simulink model "IOControls"  (R2019b)
settings: configuration reference "ConfigSet_IOControls_Reference" (kept outside this file)
model workspace (MAT data in the model file):
  SampleTime = 0.05
libraries: IOStateMachinesLib x274, SignalGeneratorsLib x1, simulink x1
(part 9 of 10)

== system IOControls/ForEachVehicle/IOControls/Non-CabControl/PneumaticControls/EPIC ==
  note: States:
      | Isolated
      | Normal
  InputControl : Inport  OutDataTypeStr=Bus: BD_IOControls_In_InputControl
  Initialise : Inport  Port=2
  Bus Selector : BusSelector  OutputSignals=Value,Mode,InitVal,InternalRequest,Inhibit
  EPIC-Toggle : IOStateMachinesLib/Toggle  InitSource=internal  InitState=InitState  OffStateValue=OffStateValue  OnStateValue=OnStateValue
      settings: SourceProductName=IO State Machines
  InputState : Outport  VectorParamsAs1DForOutWhenUnconnected=off
  wires:
  Initialise/1 -> EPIC-Toggle/4
  EPIC-Toggle/1 -> InputState/1
  Bus Selector/5 -> EPIC-Toggle/6  "<Inhibit>"
  Bus Selector/4 -> EPIC-Toggle/5  "<InternalRequest>"
  Bus Selector/3 -> EPIC-Toggle/3  "<InitVal>"
  Bus Selector/2 -> EPIC-Toggle/2  "<Mode>"
  Bus Selector/1 -> EPIC-Toggle/1  "<Value>"
  InputControl/1 -> Bus Selector/1

== system IOControls/ForEachVehicle/IOControls/Non-CabControl/PneumaticControls/Horn1IsolationCock ==
  note: States:
      | Isolated
      | Normal
  InputControl : Inport  OutDataTypeStr=Bus: BD_IOControls_In_InputControl
  Initialise : Inport  Port=2
  Bus Selector : BusSelector  OutputSignals=Value,Mode,InitVal,InternalRequest,Inhibit
  Horn1IsolationCock-Toggle : IOStateMachinesLib/Toggle  InitSource=internal  InitState=InitState  OffStateValue=OffStateValue  OnStateValue=OnStateValue
      settings: SourceProductName=IO State Machines
  InputState : Outport  VectorParamsAs1DForOutWhenUnconnected=off
  wires:
  Initialise/1 -> Horn1IsolationCock-Toggle/4
  Horn1IsolationCock-Toggle/1 -> InputState/1
  Bus Selector/5 -> Horn1IsolationCock-Toggle/6  "<Inhibit>"
  Bus Selector/4 -> Horn1IsolationCock-Toggle/5  "<InternalRequest>"
  Bus Selector/3 -> Horn1IsolationCock-Toggle/3  "<InitVal>"
  Bus Selector/2 -> Horn1IsolationCock-Toggle/2  "<Mode>"
  Bus Selector/1 -> Horn1IsolationCock-Toggle/1  "<Value>"
  InputControl/1 -> Bus Selector/1

== system IOControls/ForEachVehicle/IOControls/Non-CabControl/PneumaticControls/Horn2IsolationCock ==
  note: States:
      | Isolated
      | Normal
  InputControl : Inport  OutDataTypeStr=Bus: BD_IOControls_In_InputControl
  Initialise : Inport  Port=2
  Bus Selector : BusSelector  OutputSignals=Value,Mode,InitVal,InternalRequest,Inhibit
  Horn2IsolationCock-Toggle : IOStateMachinesLib/Toggle  InitSource=internal  InitState=InitState  OffStateValue=OffStateValue  OnStateValue=OnStateValue
      settings: SourceProductName=IO State Machines
  InputState : Outport  VectorParamsAs1DForOutWhenUnconnected=off
  wires:
  Initialise/1 -> Horn2IsolationCock-Toggle/4
  Horn2IsolationCock-Toggle/1 -> InputState/1
  Bus Selector/5 -> Horn2IsolationCock-Toggle/6  "<Inhibit>"
  Bus Selector/4 -> Horn2IsolationCock-Toggle/5  "<InternalRequest>"
  Bus Selector/3 -> Horn2IsolationCock-Toggle/3  "<InitVal>"
  Bus Selector/2 -> Horn2IsolationCock-Toggle/2  "<Mode>"
  Bus Selector/1 -> Horn2IsolationCock-Toggle/1  "<Value>"
  InputControl/1 -> Bus Selector/1

== system IOControls/ForEachVehicle/IOControls/Non-CabControl/PneumaticControls/MREPIsolationCockEnd1 ==
  note: States:
      | Isolated
      | Normal
  InputControl : Inport  OutDataTypeStr=Bus: BD_IOControls_In_InputControl
  Initialise : Inport  Port=2
  Bus Selector : BusSelector  OutputSignals=Value,Mode,InitVal,InternalRequest,Inhibit
  MREPIsolationCockEnd1-Toggle : IOStateMachinesLib/Toggle  InitSource=internal  InitState=InitState  OffStateValue=OffStateValue  OnStateValue=OnStateValue
      settings: SourceProductName=IO State Machines
  InputState : Outport  VectorParamsAs1DForOutWhenUnconnected=off
  wires:
  Initialise/1 -> MREPIsolationCockEnd1-Toggle/4
  MREPIsolationCockEnd1-Toggle/1 -> InputState/1
  Bus Selector/5 -> MREPIsolationCockEnd1-Toggle/6  "<Inhibit>"
  Bus Selector/4 -> MREPIsolationCockEnd1-Toggle/5  "<InternalRequest>"
  Bus Selector/3 -> MREPIsolationCockEnd1-Toggle/3  "<InitVal>"
  Bus Selector/2 -> MREPIsolationCockEnd1-Toggle/2  "<Mode>"
  Bus Selector/1 -> MREPIsolationCockEnd1-Toggle/1  "<Value>"
  InputControl/1 -> Bus Selector/1

== system IOControls/ForEachVehicle/IOControls/Non-CabControl/PneumaticControls/MREPIsolationCockEnd2 ==
  note: States:
      | Isolated
      | Normal
  InputControl : Inport  OutDataTypeStr=Bus: BD_IOControls_In_InputControl
  Initialise : Inport  Port=2
  Bus Selector : BusSelector  OutputSignals=Value,Mode,InitVal,InternalRequest,Inhibit
  MREPIsolationCockEnd2-Toggle : IOStateMachinesLib/Toggle  InitSource=internal  InitState=InitState  OffStateValue=OffStateValue  OnStateValue=OnStateValue
      settings: SourceProductName=IO State Machines
  InputState : Outport  VectorParamsAs1DForOutWhenUnconnected=off
  wires:
  Initialise/1 -> MREPIsolationCockEnd2-Toggle/4
  MREPIsolationCockEnd2-Toggle/1 -> InputState/1
  Bus Selector/5 -> MREPIsolationCockEnd2-Toggle/6  "<Inhibit>"
  Bus Selector/4 -> MREPIsolationCockEnd2-Toggle/5  "<InternalRequest>"
  Bus Selector/3 -> MREPIsolationCockEnd2-Toggle/3  "<InitVal>"
  Bus Selector/2 -> MREPIsolationCockEnd2-Toggle/2  "<Mode>"
  Bus Selector/1 -> MREPIsolationCockEnd2-Toggle/1  "<Value>"
  InputControl/1 -> Bus Selector/1

== system IOControls/ForEachVehicle/IOControls/Non-CabControl/PneumaticControls/MRIsolationCock ==
  note: States:
      | Isolated
      | Normal
  InputControl : Inport  OutDataTypeStr=Bus: BD_IOControls_In_InputControl
  Initialise : Inport  Port=2
  Bus Selector : BusSelector  OutputSignals=Value,Mode,InitVal,InternalRequest,Inhibit
  MRIsolationCock-Toggle : IOStateMachinesLib/Toggle  InitSource=internal  InitState=InitState  OffStateValue=OffStateValue  OnStateValue=OnStateValue
      settings: SourceProductName=IO State Machines
  InputState : Outport  VectorParamsAs1DForOutWhenUnconnected=off
  wires:
  Initialise/1 -> MRIsolationCock-Toggle/4
  MRIsolationCock-Toggle/1 -> InputState/1
  Bus Selector/5 -> MRIsolationCock-Toggle/6  "<Inhibit>"
  Bus Selector/4 -> MRIsolationCock-Toggle/5  "<InternalRequest>"
  Bus Selector/3 -> MRIsolationCock-Toggle/3  "<InitVal>"
  Bus Selector/2 -> MRIsolationCock-Toggle/2  "<Mode>"
  Bus Selector/1 -> MRIsolationCock-Toggle/1  "<Value>"
  InputControl/1 -> Bus Selector/1

== system IOControls/ForEachVehicle/IOControls/Non-CabControl/PneumaticControls/ParkBrakeIsolationCockBogie1 ==
  note: States:
      | Isolated
      | Normal
  InputControl : Inport  OutDataTypeStr=Bus: BD_IOControls_In_InputControl
  Initialise : Inport  Port=2
  Bus Selector : BusSelector  OutputSignals=Value,Mode,InitVal,InternalRequest,Inhibit
  ParkBrakeIsolationCockBogie1-Toggle : IOStateMachinesLib/Toggle  InitSource=internal  InitState=InitState  OffStateValue=OffStateValue  OnStateValue=OnStateValue
      settings: SourceProductName=IO State Machines
  InputState : Outport  VectorParamsAs1DForOutWhenUnconnected=off
  wires:
  Initialise/1 -> ParkBrakeIsolationCockBogie1-Toggle/4
  ParkBrakeIsolationCockBogie1-Toggle/1 -> InputState/1
  Bus Selector/5 -> ParkBrakeIsolationCockBogie1-Toggle/6  "<Inhibit>"
  Bus Selector/4 -> ParkBrakeIsolationCockBogie1-Toggle/5  "<InternalRequest>"
  Bus Selector/3 -> ParkBrakeIsolationCockBogie1-Toggle/3  "<InitVal>"
  Bus Selector/2 -> ParkBrakeIsolationCockBogie1-Toggle/2  "<Mode>"
  Bus Selector/1 -> ParkBrakeIsolationCockBogie1-Toggle/1  "<Value>"
  InputControl/1 -> Bus Selector/1

== system IOControls/ForEachVehicle/IOControls/Non-CabControl/PneumaticControls/ParkBrakeIsolationCockBogie2 ==
  note: States:
      | Isolated
      | Normal
  InputControl : Inport  OutDataTypeStr=Bus: BD_IOControls_In_InputControl
  Initialise : Inport  Port=2
  Bus Selector : BusSelector  OutputSignals=Value,Mode,InitVal,InternalRequest,Inhibit
  ParkBrakeIsolationCockBogie2-Toggle : IOStateMachinesLib/Toggle  InitSource=internal  InitState=InitState  OffStateValue=OffStateValue  OnStateValue=OnStateValue
      settings: SourceProductName=IO State Machines
  InputState : Outport  VectorParamsAs1DForOutWhenUnconnected=off
  wires:
  Initialise/1 -> ParkBrakeIsolationCockBogie2-Toggle/4
  ParkBrakeIsolationCockBogie2-Toggle/1 -> InputState/1
  Bus Selector/5 -> ParkBrakeIsolationCockBogie2-Toggle/6  "<Inhibit>"
  Bus Selector/4 -> ParkBrakeIsolationCockBogie2-Toggle/5  "<InternalRequest>"
  Bus Selector/3 -> ParkBrakeIsolationCockBogie2-Toggle/3  "<InitVal>"
  Bus Selector/2 -> ParkBrakeIsolationCockBogie2-Toggle/2  "<Mode>"
  Bus Selector/1 -> ParkBrakeIsolationCockBogie2-Toggle/1  "<Value>"
  InputControl/1 -> Bus Selector/1

== system IOControls/ForEachVehicle/IOControls/Non-CabControl/PneumaticControls/ParkingBrakeManualReleaseBogie1Handle1 ==
  note: States:
      | Normal
      | Pulled
  InputControl : Inport  OutDataTypeStr=Bus: BD_IOControls_In_InputControl
  Initialise : Inport  Port=2
  Bus Selector : BusSelector  OutputSignals=Value,Mode,InitVal,InternalRequest,Inhibit
  ParkingBrakeManualReleaseBogie1Handle1-Toggle : IOStateMachinesLib/Toggle  InitSource=internal  InitState=InitState  OffStateValue=OffStateValue  OnStateValue=OnStateValue
      settings: SourceProductName=IO State Machines
  InputState : Outport  VectorParamsAs1DForOutWhenUnconnected=off
  wires:
  Initialise/1 -> ParkingBrakeManualReleaseBogie1Handle1-Toggle/4
  ParkingBrakeManualReleaseBogie1Handle1-Toggle/1 -> InputState/1
  Bus Selector/5 -> ParkingBrakeManualReleaseBogie1Handle1-Toggle/6  "<Inhibit>"
  Bus Selector/4 -> ParkingBrakeManualReleaseBogie1Handle1-Toggle/5  "<InternalRequest>"
  Bus Selector/3 -> ParkingBrakeManualReleaseBogie1Handle1-Toggle/3  "<InitVal>"
  Bus Selector/2 -> ParkingBrakeManualReleaseBogie1Handle1-Toggle/2  "<Mode>"
  Bus Selector/1 -> ParkingBrakeManualReleaseBogie1Handle1-Toggle/1  "<Value>"
  InputControl/1 -> Bus Selector/1

== system IOControls/ForEachVehicle/IOControls/Non-CabControl/PneumaticControls/ParkingBrakeManualReleaseBogie1Handle2 ==
  note: States:
      | Normal
      | Pulled
  InputControl : Inport  OutDataTypeStr=Bus: BD_IOControls_In_InputControl
  Initialise : Inport  Port=2
  Bus Selector : BusSelector  OutputSignals=Value,Mode,InitVal,InternalRequest,Inhibit
  ParkingBrakeManualReleaseBogie1Handle2-Toggle : IOStateMachinesLib/Toggle  InitSource=internal  InitState=InitState  OffStateValue=OffStateValue  OnStateValue=OnStateValue
      settings: SourceProductName=IO State Machines
  InputState : Outport  VectorParamsAs1DForOutWhenUnconnected=off
  wires:
  Initialise/1 -> ParkingBrakeManualReleaseBogie1Handle2-Toggle/4
  ParkingBrakeManualReleaseBogie1Handle2-Toggle/1 -> InputState/1
  Bus Selector/5 -> ParkingBrakeManualReleaseBogie1Handle2-Toggle/6  "<Inhibit>"
  Bus Selector/4 -> ParkingBrakeManualReleaseBogie1Handle2-Toggle/5  "<InternalRequest>"
  Bus Selector/3 -> ParkingBrakeManualReleaseBogie1Handle2-Toggle/3  "<InitVal>"
  Bus Selector/2 -> ParkingBrakeManualReleaseBogie1Handle2-Toggle/2  "<Mode>"
  Bus Selector/1 -> ParkingBrakeManualReleaseBogie1Handle2-Toggle/1  "<Value>"
  InputControl/1 -> Bus Selector/1

== system IOControls/ForEachVehicle/IOControls/Non-CabControl/PneumaticControls/ParkingBrakeManualReleaseBogie2Handle1 ==
  note: States:
      | Normal
      | Pulled
  InputControl : Inport  OutDataTypeStr=Bus: BD_IOControls_In_InputControl
  Initialise : Inport  Port=2
  Bus Selector : BusSelector  OutputSignals=Value,Mode,InitVal,InternalRequest,Inhibit
  ParkingBrakeManualReleaseBogie2Handle1-Toggle : IOStateMachinesLib/Toggle  InitSource=internal  InitState=InitState  OffStateValue=OffStateValue  OnStateValue=OnStateValue
      settings: SourceProductName=IO State Machines
  InputState : Outport  VectorParamsAs1DForOutWhenUnconnected=off
  wires:
  Initialise/1 -> ParkingBrakeManualReleaseBogie2Handle1-Toggle/4
  ParkingBrakeManualReleaseBogie2Handle1-Toggle/1 -> InputState/1
  Bus Selector/5 -> ParkingBrakeManualReleaseBogie2Handle1-Toggle/6  "<Inhibit>"
  Bus Selector/4 -> ParkingBrakeManualReleaseBogie2Handle1-Toggle/5  "<InternalRequest>"
  Bus Selector/3 -> ParkingBrakeManualReleaseBogie2Handle1-Toggle/3  "<InitVal>"
  Bus Selector/2 -> ParkingBrakeManualReleaseBogie2Handle1-Toggle/2  "<Mode>"
  Bus Selector/1 -> ParkingBrakeManualReleaseBogie2Handle1-Toggle/1  "<Value>"
  InputControl/1 -> Bus Selector/1

== system IOControls/ForEachVehicle/IOControls/Non-CabControl/PneumaticControls/ParkingBrakeManualReleaseBogie2Handle2 ==
  note: States:
      | Normal
      | Pulled
  InputControl : Inport  OutDataTypeStr=Bus: BD_IOControls_In_InputControl
  Initialise : Inport  Port=2
  Bus Selector : BusSelector  OutputSignals=Value,Mode,InitVal,InternalRequest,Inhibit
  ParkingBrakeManualReleaseBogie2Handle2-Toggle : IOStateMachinesLib/Toggle  InitSource=internal  InitState=InitState  OffStateValue=OffStateValue  OnStateValue=OnStateValue
      settings: SourceProductName=IO State Machines
  InputState : Outport  VectorParamsAs1DForOutWhenUnconnected=off
  wires:
  Initialise/1 -> ParkingBrakeManualReleaseBogie2Handle2-Toggle/4
  ParkingBrakeManualReleaseBogie2Handle2-Toggle/1 -> InputState/1
  Bus Selector/5 -> ParkingBrakeManualReleaseBogie2Handle2-Toggle/6  "<Inhibit>"
  Bus Selector/4 -> ParkingBrakeManualReleaseBogie2Handle2-Toggle/5  "<InternalRequest>"
  Bus Selector/3 -> ParkingBrakeManualReleaseBogie2Handle2-Toggle/3  "<InitVal>"
  Bus Selector/2 -> ParkingBrakeManualReleaseBogie2Handle2-Toggle/2  "<Mode>"
  Bus Selector/1 -> ParkingBrakeManualReleaseBogie2Handle2-Toggle/1  "<Value>"
  InputControl/1 -> Bus Selector/1

== system IOControls/ForEachVehicle/IOControls/Non-CabControl/PneumaticControls/SR ==
  note: States:
      | Isolated
      | Normal
  InputControl : Inport  OutDataTypeStr=Bus: BD_IOControls_In_InputControl
  Initialise : Inport  Port=2
  Bus Selector : BusSelector  OutputSignals=Value,Mode,InitVal,InternalRequest,Inhibit
  SR-Toggle : IOStateMachinesLib/Toggle  InitSource=internal  InitState=InitState  OffStateValue=OffStateValue  OnStateValue=OnStateValue
      settings: SourceProductName=IO State Machines
  InputState : Outport  VectorParamsAs1DForOutWhenUnconnected=off
  wires:
  Initialise/1 -> SR-Toggle/4
  SR-Toggle/1 -> InputState/1
  Bus Selector/5 -> SR-Toggle/6  "<Inhibit>"
  Bus Selector/4 -> SR-Toggle/5  "<InternalRequest>"
  Bus Selector/3 -> SR-Toggle/3  "<InitVal>"
  Bus Selector/2 -> SR-Toggle/2  "<Mode>"
  Bus Selector/1 -> SR-Toggle/1  "<Value>"
  InputControl/1 -> Bus Selector/1

== system IOControls/ForEachVehicle/IOControls/Non-CabControl/PneumaticControls/UncouplingCock ==
  note: States:
      | Isolated
      | Normal
  InputControl : Inport  OutDataTypeStr=Bus: BD_IOControls_In_InputControl
  Initialise : Inport  Port=2
  Bus Selector : BusSelector  OutputSignals=Value,Mode,InitVal,InternalRequest,Inhibit
  UncouplingCock-Toggle : IOStateMachinesLib/Toggle  InitSource=internal  InitState=InitState  OffStateValue=OffStateValue  OnStateValue=OnStateValue
      settings: SourceProductName=IO State Machines
  InputState : Outport  VectorParamsAs1DForOutWhenUnconnected=off
  wires:
  Initialise/1 -> UncouplingCock-Toggle/4
  UncouplingCock-Toggle/1 -> InputState/1
  Bus Selector/5 -> UncouplingCock-Toggle/6  "<Inhibit>"
  Bus Selector/4 -> UncouplingCock-Toggle/5  "<InternalRequest>"
  Bus Selector/3 -> UncouplingCock-Toggle/3  "<InitVal>"
  Bus Selector/2 -> UncouplingCock-Toggle/2  "<Mode>"
  Bus Selector/1 -> UncouplingCock-Toggle/1  "<Value>"
  InputControl/1 -> Bus Selector/1

== system IOControls/ForEachVehicle/IOControls/CabControl/DriverDesk/MasterController/ControlKey ==
  note: States:
      | Off
      | On
  InputControl : Inport  OutDataTypeStr=Bus: BD_IOControls_In_InputControl
  Initialise : Inport  Port=2
  Bus Selector : BusSelector  OutputSignals=Value,Mode,InitVal,InternalRequest,Inhibit
  ControlKey-Toggle : IOStateMachinesLib/Toggle  InitSource=internal  InitState=InitState  OffStateValue=OffStateValue  OnStateValue=OnStateValue
      settings: SourceProductName=IO State Machines
  InputState : Outport  VectorParamsAs1DForOutWhenUnconnected=off
  wires:
  Initialise/1 -> ControlKey-Toggle/4
  ControlKey-Toggle/1 -> InputState/1
  Bus Selector/5 -> ControlKey-Toggle/6  "<Inhibit>"
  Bus Selector/4 -> ControlKey-Toggle/5  "<InternalRequest>"
  Bus Selector/3 -> ControlKey-Toggle/3  "<InitVal>"
  Bus Selector/2 -> ControlKey-Toggle/2  "<Mode>"
  Bus Selector/1 -> ControlKey-Toggle/1  "<Value>"
  InputControl/1 -> Bus Selector/1

== system IOControls/ForEachVehicle/IOControls/CabControl/DriverDesk/MasterController/DeadmanSafetyDevice ==
  note: States:
      | Off
      | On
  InputControl : Inport  OutDataTypeStr=Bus: BD_IOControls_In_InputControl
  Initialise : Inport  Port=2
  Bus Selector : BusSelector  OutputSignals=Value,Mode,InitVal,InternalRequest,Inhibit
  DeadmanSafetyDevice-Toggle : IOStateMachinesLib/Toggle  InitSource=internal  InitState=InitState  OffStateValue=OffStateValue  OnStateValue=OnStateValue
      settings: SourceProductName=IO State Machines
  InputState : Outport  VectorParamsAs1DForOutWhenUnconnected=off
  wires:
  Initialise/1 -> DeadmanSafetyDevice-Toggle/4
  DeadmanSafetyDevice-Toggle/1 -> InputState/1
  Bus Selector/5 -> DeadmanSafetyDevice-Toggle/6  "<Inhibit>"
  Bus Selector/4 -> DeadmanSafetyDevice-Toggle/5  "<InternalRequest>"
  Bus Selector/3 -> DeadmanSafetyDevice-Toggle/3  "<InitVal>"
  Bus Selector/2 -> DeadmanSafetyDevice-Toggle/2  "<Mode>"
  Bus Selector/1 -> DeadmanSafetyDevice-Toggle/1  "<Value>"
  InputControl/1 -> Bus Selector/1

== system IOControls/ForEachVehicle/IOControls/CabControl/DriverDesk/MasterController/MasterControllerHandle ==
  note: States:
      | EB
      | Bmax
      | Bmin
      | Off
      | Pmin
      | Pmin
  InputControl : Inport  OutDataTypeStr=Bus: BD_IOControls_In_InputControl
  Initialise : Inport  Port=2
  Bus Selector : BusSelector  OutputSignals=Value,Mode,InitVal,InternalRequest,Inhibit
  MasterControllerHandle-Increment : IOStateMachinesLib/Increment  InitSource=internal  InitState=InitState  ControlStates=ControlStates
      settings: SourceProductName=IO State Machines
  InputState : Outport  VectorParamsAs1DForOutWhenUnconnected=off
  wires:
  Initialise/1 -> MasterControllerHandle-Increment/4
  MasterControllerHandle-Increment/1 -> InputState/1
  Bus Selector/5 -> MasterControllerHandle-Increment/6  "<Inhibit>"
  Bus Selector/4 -> MasterControllerHandle-Increment/5  "<InternalRequest>"
  Bus Selector/3 -> MasterControllerHandle-Increment/3  "<InitVal>"
  Bus Selector/2 -> MasterControllerHandle-Increment/2  "<Mode>"
  Bus Selector/1 -> MasterControllerHandle-Increment/1  "<Value>"
  InputControl/1 -> Bus Selector/1

== system IOControls/ForEachVehicle/IOControls/CabControl/DriverDesk/MasterController/ModeSelector ==
  note: States:
      | Off UTO
      | Reverse
      | Standby
      | Forword
      | ATP
      | ATO
  InputControl : Inport  OutDataTypeStr=Bus: BD_IOControls_In_InputControl
  Initialise : Inport  Port=2
  Bus Selector : BusSelector  OutputSignals=Value,Mode,InitVal,InternalRequest,Inhibit
  ModeSelector-Increment : IOStateMachinesLib/Increment  InitSource=internal  InitState=InitState  ControlStates=ControlStates
      settings: SourceProductName=IO State Machines
  InputState : Outport  VectorParamsAs1DForOutWhenUnconnected=off
  wires:
  Initialise/1 -> ModeSelector-Increment/4
  ModeSelector-Increment/1 -> InputState/1
  Bus Selector/5 -> ModeSelector-Increment/6  "<Inhibit>"
  Bus Selector/4 -> ModeSelector-Increment/5  "<InternalRequest>"
  Bus Selector/3 -> ModeSelector-Increment/3  "<InitVal>"
  Bus Selector/2 -> ModeSelector-Increment/2  "<Mode>"
  Bus Selector/1 -> ModeSelector-Increment/1  "<Value>"
  InputControl/1 -> Bus Selector/1

== system IOControls/ForEachVehicle/IOControls/CabControl/DriverDesk/OperatingPanel1/CabConsoleLightPB ==
  note: States:
      | Off
      | On
  InputControl : Inport  OutDataTypeStr=Bus: BD_IOControls_In_InputControl
  Initialise : Inport  Port=2
  Bus Selector : BusSelector  OutputSignals=Value,Mode,InitVal,InternalRequest,Inhibit
  CabConsoleLightPB-Toggle : IOStateMachinesLib/Toggle  InitSource=internal  InitState=InitState  OffStateValue=OffStateValue  OnStateValue=OnStateValue
      settings: SourceProductName=IO State Machines
  InputState : Outport  VectorParamsAs1DForOutWhenUnconnected=off
  wires:
  Initialise/1 -> CabConsoleLightPB-Toggle/4
  CabConsoleLightPB-Toggle/1 -> InputState/1
  Bus Selector/5 -> CabConsoleLightPB-Toggle/6  "<Inhibit>"
  Bus Selector/4 -> CabConsoleLightPB-Toggle/5  "<InternalRequest>"
  Bus Selector/3 -> CabConsoleLightPB-Toggle/3  "<InitVal>"
  Bus Selector/2 -> CabConsoleLightPB-Toggle/2  "<Mode>"
  Bus Selector/1 -> CabConsoleLightPB-Toggle/1  "<Value>"
  InputControl/1 -> Bus Selector/1

== system IOControls/ForEachVehicle/IOControls/CabControl/DriverDesk/OperatingPanel1/CabMainLightPB ==
  note: States:
      | Off
      | On
  InputControl : Inport  OutDataTypeStr=Bus: BD_IOControls_In_InputControl
  Initialise : Inport  Port=2
  Bus Selector : BusSelector  OutputSignals=Value,Mode,InitVal,InternalRequest,Inhibit
  CabMainLightPB-Toggle : IOStateMachinesLib/Toggle  InitSource=internal  InitState=InitState  OffStateValue=OffStateValue  OnStateValue=OnStateValue
      settings: SourceProductName=IO State Machines
  InputState : Outport  VectorParamsAs1DForOutWhenUnconnected=off
  wires:
  Initialise/1 -> CabMainLightPB-Toggle/4
  CabMainLightPB-Toggle/1 -> InputState/1
  Bus Selector/5 -> CabMainLightPB-Toggle/6  "<Inhibit>"
  Bus Selector/4 -> CabMainLightPB-Toggle/5  "<InternalRequest>"
  Bus Selector/3 -> CabMainLightPB-Toggle/3  "<InitVal>"
  Bus Selector/2 -> CabMainLightPB-Toggle/2  "<Mode>"
  Bus Selector/1 -> CabMainLightPB-Toggle/1  "<Value>"
  InputControl/1 -> Bus Selector/1

== system IOControls/ForEachVehicle/IOControls/CabControl/DriverDesk/OperatingPanel1/DoorCloseAnnouncementPB ==
  note: States:
      | Off
      | On
  InputControl : Inport  OutDataTypeStr=Bus: BD_IOControls_In_InputControl
  Initialise : Inport  Port=2
  Bus Selector : BusSelector  OutputSignals=Value,Mode,InitVal,InternalRequest,Inhibit
  DoorCloseAnnouncementPB-Momentary : IOStateMachinesLib/Momentary  InitSource=internal  InitState=InitState
      settings: SourceProductName=IO State Machines
  InputState : Outport  VectorParamsAs1DForOutWhenUnconnected=off
  wires:
  Initialise/1 -> DoorCloseAnnouncementPB-Momentary/4
  DoorCloseAnnouncementPB-Momentary/1 -> InputState/1
  Bus Selector/5 -> DoorCloseAnnouncementPB-Momentary/6  "<Inhibit>"
  Bus Selector/4 -> DoorCloseAnnouncementPB-Momentary/5  "<InternalRequest>"
  Bus Selector/3 -> DoorCloseAnnouncementPB-Momentary/3  "<InitVal>"
  Bus Selector/2 -> DoorCloseAnnouncementPB-Momentary/2  "<Mode>"
  Bus Selector/1 -> DoorCloseAnnouncementPB-Momentary/1  "<Value>"
  InputControl/1 -> Bus Selector/1

== system IOControls/ForEachVehicle/IOControls/CabControl/DriverDesk/OperatingPanel1/DoorProvenLoopCutoutPB ==
  note: States:
      | Off
      | On
  InputControl : Inport  OutDataTypeStr=Bus: BD_IOControls_In_InputControl
  Initialise : Inport  Port=2
  Bus Selector : BusSelector  OutputSignals=Value,Mode,InitVal,InternalRequest,Inhibit
  DoorProvenLoopCutoutPB-Momentary : IOStateMachinesLib/Momentary  InitSource=internal  InitState=InitState
      settings: SourceProductName=IO State Machines
  InputState : Outport  VectorParamsAs1DForOutWhenUnconnected=off
  wires:
  Initialise/1 -> DoorProvenLoopCutoutPB-Momentary/4
  DoorProvenLoopCutoutPB-Momentary/1 -> InputState/1
  Bus Selector/5 -> DoorProvenLoopCutoutPB-Momentary/6  "<Inhibit>"
  Bus Selector/4 -> DoorProvenLoopCutoutPB-Momentary/5  "<InternalRequest>"
  Bus Selector/3 -> DoorProvenLoopCutoutPB-Momentary/3  "<InitVal>"
  Bus Selector/2 -> DoorProvenLoopCutoutPB-Momentary/2  "<Mode>"
  Bus Selector/1 -> DoorProvenLoopCutoutPB-Momentary/1  "<Value>"
  InputControl/1 -> Bus Selector/1

== system IOControls/ForEachVehicle/IOControls/CabControl/DriverDesk/OperatingPanel1/EmergencyBrakePB ==
  note: States:
      | Off
      | On
  InputControl : Inport  OutDataTypeStr=Bus: BD_IOControls_In_InputControl
  Initialise : Inport  Port=2
  Bus Selector : BusSelector  OutputSignals=Value,Mode,InitVal,InternalRequest,Inhibit
  EmergencyBrakePB-Toggle : IOStateMachinesLib/Toggle  InitSource=internal  InitState=InitState  OffStateValue=OffStateValue  OnStateValue=OnStateValue
      settings: SourceProductName=IO State Machines
  InputState : Outport  VectorParamsAs1DForOutWhenUnconnected=off
  wires:
  Initialise/1 -> EmergencyBrakePB-Toggle/4
  EmergencyBrakePB-Toggle/1 -> InputState/1
  Bus Selector/5 -> EmergencyBrakePB-Toggle/6  "<Inhibit>"
  Bus Selector/4 -> EmergencyBrakePB-Toggle/5  "<InternalRequest>"
  Bus Selector/3 -> EmergencyBrakePB-Toggle/3  "<InitVal>"
  Bus Selector/2 -> EmergencyBrakePB-Toggle/2  "<Mode>"
  Bus Selector/1 -> EmergencyBrakePB-Toggle/1  "<Value>"
  InputControl/1 -> Bus Selector/1

== system IOControls/ForEachVehicle/IOControls/CabControl/DriverDesk/OperatingPanel1/HornPB ==
  note: States:
      | Off
      | On
  InputControl : Inport  OutDataTypeStr=Bus: BD_IOControls_In_InputControl
  Initialise : Inport  Port=2
  Bus Selector : BusSelector  OutputSignals=Value,Mode,InitVal,InternalRequest,Inhibit
  HornPB-Momentary : IOStateMachinesLib/Momentary  InitSource=internal  InitState=InitState
      settings: SourceProductName=IO State Machines
  InputState : Outport  VectorParamsAs1DForOutWhenUnconnected=off
  wires:
  Initialise/1 -> HornPB-Momentary/4
  HornPB-Momentary/1 -> InputState/1
  Bus Selector/5 -> HornPB-Momentary/6  "<Inhibit>"
  Bus Selector/4 -> HornPB-Momentary/5  "<InternalRequest>"
  Bus Selector/3 -> HornPB-Momentary/3  "<InitVal>"
  Bus Selector/2 -> HornPB-Momentary/2  "<Mode>"
  Bus Selector/1 -> HornPB-Momentary/1  "<Value>"
  InputControl/1 -> Bus Selector/1

== system IOControls/ForEachVehicle/IOControls/CabControl/DriverDesk/OperatingPanel1/LeftDoorClosePBOperatingPanel1 ==
  note: States:
      | Off
      | On
  InputControl : Inport  OutDataTypeStr=Bus: BD_IOControls_In_InputControl
  Initialise : Inport  Port=2
  Bus Selector : BusSelector  OutputSignals=Value,Mode,InitVal,InternalRequest,Inhibit
  LeftDoorClosePBOperatingPanel1-Momentary : IOStateMachinesLib/Momentary  InitSource=internal  InitState=InitState
      settings: SourceProductName=IO State Machines
  InputState : Outport  VectorParamsAs1DForOutWhenUnconnected=off
  wires:
  Initialise/1 -> LeftDoorClosePBOperatingPanel1-Momentary/4
  LeftDoorClosePBOperatingPanel1-Momentary/1 -> InputState/1
  Bus Selector/5 -> LeftDoorClosePBOperatingPanel1-Momentary/6  "<Inhibit>"
  Bus Selector/4 -> LeftDoorClosePBOperatingPanel1-Momentary/5  "<InternalRequest>"
  Bus Selector/3 -> LeftDoorClosePBOperatingPanel1-Momentary/3  "<InitVal>"
  Bus Selector/2 -> LeftDoorClosePBOperatingPanel1-Momentary/2  "<Mode>"
  Bus Selector/1 -> LeftDoorClosePBOperatingPanel1-Momentary/1  "<Value>"
  InputControl/1 -> Bus Selector/1

== system IOControls/ForEachVehicle/IOControls/CabControl/DriverDesk/OperatingPanel1/LeftDoorOpenPBOperatingPanel1 ==
  note: States:
      | Off
      | On
  InputControl : Inport  OutDataTypeStr=Bus: BD_IOControls_In_InputControl
  Initialise : Inport  Port=2
  Bus Selector : BusSelector  OutputSignals=Value,Mode,InitVal,InternalRequest,Inhibit
  LeftDoorOpenPBOperatingPanel1-Momentary : IOStateMachinesLib/Momentary  InitSource=internal  InitState=InitState
      settings: SourceProductName=IO State Machines
  InputState : Outport  VectorParamsAs1DForOutWhenUnconnected=off
  wires:
  Initialise/1 -> LeftDoorOpenPBOperatingPanel1-Momentary/4
  LeftDoorOpenPBOperatingPanel1-Momentary/1 -> InputState/1
  Bus Selector/5 -> LeftDoorOpenPBOperatingPanel1-Momentary/6  "<Inhibit>"
  Bus Selector/4 -> LeftDoorOpenPBOperatingPanel1-Momentary/5  "<InternalRequest>"
  Bus Selector/3 -> LeftDoorOpenPBOperatingPanel1-Momentary/3  "<InitVal>"
  Bus Selector/2 -> LeftDoorOpenPBOperatingPanel1-Momentary/2  "<Mode>"
  Bus Selector/1 -> LeftDoorOpenPBOperatingPanel1-Momentary/1  "<Value>"
  InputControl/1 -> Bus Selector/1

== system IOControls/ForEachVehicle/IOControls/CabControl/DriverDesk/OperatingPanel1/ParkingBrakeOffSwitch ==
  note: States:
      | Off
      | On
  InputControl : Inport  OutDataTypeStr=Bus: BD_IOControls_In_InputControl
  Initialise : Inport  Port=2
  Bus Selector : BusSelector  OutputSignals=Value,Mode,InitVal,InternalRequest,Inhibit
  ParkingBrakeOffSwitch-Momentary : IOStateMachinesLib/Momentary  InitSource=internal  InitState=InitState
      settings: SourceProductName=IO State Machines
  InputState : Outport  VectorParamsAs1DForOutWhenUnconnected=off
  wires:
  Initialise/1 -> ParkingBrakeOffSwitch-Momentary/4
  ParkingBrakeOffSwitch-Momentary/1 -> InputState/1
  Bus Selector/5 -> ParkingBrakeOffSwitch-Momentary/6  "<Inhibit>"
  Bus Selector/4 -> ParkingBrakeOffSwitch-Momentary/5  "<InternalRequest>"
  Bus Selector/3 -> ParkingBrakeOffSwitch-Momentary/3  "<InitVal>"
  Bus Selector/2 -> ParkingBrakeOffSwitch-Momentary/2  "<Mode>"
  Bus Selector/1 -> ParkingBrakeOffSwitch-Momentary/1  "<Value>"
  InputControl/1 -> Bus Selector/1

== system IOControls/ForEachVehicle/IOControls/CabControl/DriverDesk/OperatingPanel1/ParkingBrakeOnSwitch ==
  note: States:
      | Off
      | On
  InputControl : Inport  OutDataTypeStr=Bus: BD_IOControls_In_InputControl
  Initialise : Inport  Port=2
  Bus Selector : BusSelector  OutputSignals=Value,Mode,InitVal,InternalRequest,Inhibit
  ParkingBrakeOnSwitch-Momentary : IOStateMachinesLib/Momentary  InitSource=internal  InitState=InitState
      settings: SourceProductName=IO State Machines
  InputState : Outport  VectorParamsAs1DForOutWhenUnconnected=off
  wires:
  Initialise/1 -> ParkingBrakeOnSwitch-Momentary/4
  ParkingBrakeOnSwitch-Momentary/1 -> InputState/1
  Bus Selector/5 -> ParkingBrakeOnSwitch-Momentary/6  "<Inhibit>"
  Bus Selector/4 -> ParkingBrakeOnSwitch-Momentary/5  "<InternalRequest>"
  Bus Selector/3 -> ParkingBrakeOnSwitch-Momentary/3  "<InitVal>"
  Bus Selector/2 -> ParkingBrakeOnSwitch-Momentary/2  "<Mode>"
  Bus Selector/1 -> ParkingBrakeOnSwitch-Momentary/1  "<Value>"
  InputControl/1 -> Bus Selector/1

== system IOControls/ForEachVehicle/IOControls/CabControl/DriverDesk/OperatingPanel1/RightDoorClosePBOperatingPanel1 ==
  note: States:
      | Off
      | On
  InputControl : Inport  OutDataTypeStr=Bus: BD_IOControls_In_InputControl
  Initialise : Inport  Port=2
  Bus Selector : BusSelector  OutputSignals=Value,Mode,InitVal,InternalRequest,Inhibit
  RightDoorClosePBOperatingPanel1-Momentary : IOStateMachinesLib/Momentary  InitSource=internal  InitState=InitState
      settings: SourceProductName=IO State Machines
  InputState : Outport  VectorParamsAs1DForOutWhenUnconnected=off
  wires:
  Initialise/1 -> RightDoorClosePBOperatingPanel1-Momentary/4
  RightDoorClosePBOperatingPanel1-Momentary/1 -> InputState/1
  Bus Selector/5 -> RightDoorClosePBOperatingPanel1-Momentary/6  "<Inhibit>"
  Bus Selector/4 -> RightDoorClosePBOperatingPanel1-Momentary/5  "<InternalRequest>"
  Bus Selector/3 -> RightDoorClosePBOperatingPanel1-Momentary/3  "<InitVal>"
  Bus Selector/2 -> RightDoorClosePBOperatingPanel1-Momentary/2  "<Mode>"
  Bus Selector/1 -> RightDoorClosePBOperatingPanel1-Momentary/1  "<Value>"
  InputControl/1 -> Bus Selector/1

== system IOControls/ForEachVehicle/IOControls/CabControl/DriverDesk/OperatingPanel1/RightDoorOpenPBOperatingPanel1 ==
  note: States:
      | Off
      | On
  InputControl : Inport  OutDataTypeStr=Bus: BD_IOControls_In_InputControl
  Initialise : Inport  Port=2
  Bus Selector : BusSelector  OutputSignals=Value,Mode,InitVal,InternalRequest,Inhibit
  RightDoorOpenPBOperatingPanel1-Momentary : IOStateMachinesLib/Momentary  InitSource=internal  InitState=InitState
      settings: SourceProductName=IO State Machines
  InputState : Outport  VectorParamsAs1DForOutWhenUnconnected=off
  wires:
  Initialise/1 -> RightDoorOpenPBOperatingPanel1-Momentary/4
  RightDoorOpenPBOperatingPanel1-Momentary/1 -> InputState/1
  Bus Selector/5 -> RightDoorOpenPBOperatingPanel1-Momentary/6  "<Inhibit>"
  Bus Selector/4 -> RightDoorOpenPBOperatingPanel1-Momentary/5  "<InternalRequest>"
  Bus Selector/3 -> RightDoorOpenPBOperatingPanel1-Momentary/3  "<InitVal>"
  Bus Selector/2 -> RightDoorOpenPBOperatingPanel1-Momentary/2  "<Mode>"
  Bus Selector/1 -> RightDoorOpenPBOperatingPanel1-Momentary/1  "<Value>"
  InputControl/1 -> Bus Selector/1

== system IOControls/ForEachVehicle/IOControls/CabControl/DriverDesk/OperatingPanel3/ATOStartPB ==
  note: States:
      | Off
      | On
  InputControl : Inport  OutDataTypeStr=Bus: BD_IOControls_In_InputControl
  Initialise : Inport  Port=2
  ATOStartPB-Momentary : IOStateMachinesLib/Momentary  InitSource=internal  InitState=InitState
      settings: SourceProductName=IO State Machines
  Bus Selector : BusSelector  OutputSignals=Value,Mode,InitVal,InternalRequest,Inhibit
  InputState : Outport  VectorParamsAs1DForOutWhenUnconnected=off
  wires:
  Initialise/1 -> ATOStartPB-Momentary/4
  ATOStartPB-Momentary/1 -> InputState/1
  Bus Selector/5 -> ATOStartPB-Momentary/6  "<Inhibit>"
  Bus Selector/4 -> ATOStartPB-Momentary/5  "<InternalRequest>"
  Bus Selector/3 -> ATOStartPB-Momentary/3  "<InitVal>"
  Bus Selector/2 -> ATOStartPB-Momentary/2  "<Mode>"
  Bus Selector/1 -> ATOStartPB-Momentary/1  "<Value>"
  InputControl/1 -> Bus Selector/1

== system IOControls/ForEachVehicle/IOControls/CabControl/DriverDesk/OperatingPanel3/EmergencyBrakeResetPB ==
  note: States:
      | Off
      | On
  InputControl : Inport  OutDataTypeStr=Bus: BD_IOControls_In_InputControl
  Initialise : Inport  Port=2
  Bus Selector : BusSelector  OutputSignals=Value,Mode,InitVal,InternalRequest,Inhibit
  EmergencyBrakeResetPB-Momentary : IOStateMachinesLib/Momentary  InitSource=internal  InitState=InitState
      settings: SourceProductName=IO State Machines
  InputState : Outport  VectorParamsAs1DForOutWhenUnconnected=off
  wires:
  Initialise/1 -> EmergencyBrakeResetPB-Momentary/4
  EmergencyBrakeResetPB-Momentary/1 -> InputState/1
  Bus Selector/5 -> EmergencyBrakeResetPB-Momentary/6  "<Inhibit>"
  Bus Selector/4 -> EmergencyBrakeResetPB-Momentary/5  "<InternalRequest>"
  Bus Selector/3 -> EmergencyBrakeResetPB-Momentary/3  "<InitVal>"
  Bus Selector/2 -> EmergencyBrakeResetPB-Momentary/2  "<Mode>"
  Bus Selector/1 -> EmergencyBrakeResetPB-Momentary/1  "<Value>"
  InputControl/1 -> Bus Selector/1

== system IOControls/ForEachVehicle/IOControls/CabControl/DriverDesk/OperatingPanel3/ROSPB ==
  note: States:
      | Off
      | On
  InputControl : Inport  OutDataTypeStr=Bus: BD_IOControls_In_InputControl
  Initialise : Inport  Port=2
  Bus Selector : BusSelector  OutputSignals=Value,Mode,InitVal,InternalRequest,Inhibit
  ROSPB-Momentary : IOStateMachinesLib/Momentary  InitSource=internal  InitState=InitState
      settings: SourceProductName=IO State Machines
  InputState : Outport  VectorParamsAs1DForOutWhenUnconnected=off
  wires:
  Initialise/1 -> ROSPB-Momentary/4
  ROSPB-Momentary/1 -> InputState/1
  Bus Selector/5 -> ROSPB-Momentary/6  "<Inhibit>"
  Bus Selector/4 -> ROSPB-Momentary/5  "<InternalRequest>"
  Bus Selector/3 -> ROSPB-Momentary/3  "<InitVal>"
  Bus Selector/2 -> ROSPB-Momentary/2  "<Mode>"
  Bus Selector/1 -> ROSPB-Momentary/1  "<Value>"
  InputControl/1 -> Bus Selector/1

== system IOControls/ForEachVehicle/IOControls/CabControl/DriverDesk/OperatingPanel3/UTOPB ==
  note: States:
      | Off
      | On
  InputControl : Inport  OutDataTypeStr=Bus: BD_IOControls_In_InputControl
  Initialise : Inport  Port=2
  Bus Selector : BusSelector  OutputSignals=Value,Mode,InitVal,InternalRequest,Inhibit
  UTOPB-Momentary : IOStateMachinesLib/Momentary  InitSource=internal  InitState=InitState
      settings: SourceProductName=IO State Machines
  InputState : Outport  VectorParamsAs1DForOutWhenUnconnected=off
  wires:
  Initialise/1 -> UTOPB-Momentary/4
  UTOPB-Momentary/1 -> InputState/1
  Bus Selector/5 -> UTOPB-Momentary/6  "<Inhibit>"
  Bus Selector/4 -> UTOPB-Momentary/5  "<InternalRequest>"
  Bus Selector/3 -> UTOPB-Momentary/3  "<InitVal>"
  Bus Selector/2 -> UTOPB-Momentary/2  "<Mode>"
  Bus Selector/1 -> UTOPB-Momentary/1  "<Value>"
  InputControl/1 -> Bus Selector/1

== system IOControls/ForEachVehicle/IOControls/CabControl/DriverDeskLeft/OperatingPanel2/BrakeLoopCutoutSS ==
  note: States:
      | Normal
      | Cutout
  InputControl : Inport  OutDataTypeStr=Bus: BD_IOControls_In_InputControl
  Initialise : Inport  Port=2
  BrakeLoopCutoutSS-Toggle : IOStateMachinesLib/Toggle  InitSource=internal  InitState=InitState  OffStateValue=OffStateValue  OnStateValue=OnStateValue
      settings: SourceProductName=IO State Machines
  Bus Selector : BusSelector  OutputSignals=Value,Mode,InitVal,InternalRequest,Inhibit
  InputState : Outport  VectorParamsAs1DForOutWhenUnconnected=off
  wires:
  Initialise/1 -> BrakeLoopCutoutSS-Toggle/4
  BrakeLoopCutoutSS-Toggle/1 -> InputState/1
  Bus Selector/5 -> BrakeLoopCutoutSS-Toggle/6  "<Inhibit>"
  Bus Selector/4 -> BrakeLoopCutoutSS-Toggle/5  "<InternalRequest>"
  Bus Selector/3 -> BrakeLoopCutoutSS-Toggle/3  "<InitVal>"
  Bus Selector/2 -> BrakeLoopCutoutSS-Toggle/2  "<Mode>"
  Bus Selector/1 -> BrakeLoopCutoutSS-Toggle/1  "<Value>"
  InputControl/1 -> Bus Selector/1

== system IOControls/ForEachVehicle/IOControls/CabControl/DriverDeskLeft/OperatingPanel2/CallOnLightPB ==
  note: States:
      | Off
      | On
  InputControl : Inport  OutDataTypeStr=Bus: BD_IOControls_In_InputControl
  Initialise : Inport  Port=2
  Bus Selector : BusSelector  OutputSignals=Value,Mode,InitVal,InternalRequest,Inhibit
  CallOnLightPB-Toggle : IOStateMachinesLib/Toggle  InitSource=internal  InitState=InitState  OffStateValue=OffStateValue  OnStateValue=OnStateValue
      settings: SourceProductName=IO State Machines
  InputState : Outport  VectorParamsAs1DForOutWhenUnconnected=off
  wires:
  Initialise/1 -> CallOnLightPB-Toggle/4
  CallOnLightPB-Toggle/1 -> InputState/1
  Bus Selector/5 -> CallOnLightPB-Toggle/6  "<Inhibit>"
  Bus Selector/4 -> CallOnLightPB-Toggle/5  "<InternalRequest>"
  Bus Selector/3 -> CallOnLightPB-Toggle/3  "<InitVal>"
  Bus Selector/2 -> CallOnLightPB-Toggle/2  "<Mode>"
  Bus Selector/1 -> CallOnLightPB-Toggle/1  "<Value>"
  InputControl/1 -> Bus Selector/1

== system IOControls/ForEachVehicle/IOControls/CabControl/DriverDeskLeft/OperatingPanel2/DeadmanBypassSwitch ==
  note: States:
      | Normal
      | Cutout
  InputControl : Inport  OutDataTypeStr=Bus: BD_IOControls_In_InputControl
  Initialise : Inport  Port=2
  Bus Selector : BusSelector  OutputSignals=Value,Mode,InitVal,InternalRequest,Inhibit
  DeadmanBypassSwitch-Toggle : IOStateMachinesLib/Toggle  InitSource=internal  InitState=InitState  OffStateValue=OffStateValue  OnStateValue=OnStateValue
      settings: SourceProductName=IO State Machines
  InputState : Outport  VectorParamsAs1DForOutWhenUnconnected=off
  wires:
  Initialise/1 -> DeadmanBypassSwitch-Toggle/4
  DeadmanBypassSwitch-Toggle/1 -> InputState/1
  Bus Selector/5 -> DeadmanBypassSwitch-Toggle/6  "<Inhibit>"
  Bus Selector/4 -> DeadmanBypassSwitch-Toggle/5  "<InternalRequest>"
  Bus Selector/3 -> DeadmanBypassSwitch-Toggle/3  "<InitVal>"
  Bus Selector/2 -> DeadmanBypassSwitch-Toggle/2  "<Mode>"
  Bus Selector/1 -> DeadmanBypassSwitch-Toggle/1  "<Value>"
  InputControl/1 -> Bus Selector/1

== system IOControls/ForEachVehicle/IOControls/CabControl/DriverDeskLeft/OperatingPanel2/HeadLightSwitch ==
  note: States:
      | Off
      | Low
      | High
  InputControl : Inport  OutDataTypeStr=Bus: BD_IOControls_In_InputControl
  Initialise : Inport  Port=2
  Bus Selector : BusSelector  OutputSignals=Value,Mode,InitVal,InternalRequest,Inhibit
  HeadLightSwitch-Increment : IOStateMachinesLib/Increment  InitSource=internal  InitState=InitState  ControlStates=ControlStates
      settings: SourceProductName=IO State Machines
  InputState : Outport  VectorParamsAs1DForOutWhenUnconnected=off
  wires:
  Initialise/1 -> HeadLightSwitch-Increment/4
  HeadLightSwitch-Increment/1 -> InputState/1
  Bus Selector/5 -> HeadLightSwitch-Increment/6  "<Inhibit>"
  Bus Selector/4 -> HeadLightSwitch-Increment/5  "<InternalRequest>"
  Bus Selector/3 -> HeadLightSwitch-Increment/3  "<InitVal>"
  Bus Selector/2 -> HeadLightSwitch-Increment/2  "<Mode>"
  Bus Selector/1 -> HeadLightSwitch-Increment/1  "<Value>"
  InputControl/1 -> Bus Selector/1

== system IOControls/ForEachVehicle/IOControls/CabControl/DriverDeskLeft/OperatingPanel2/LIMPHomePB ==
  note: States:
      | Off
      | On
  InputControl : Inport  OutDataTypeStr=Bus: BD_IOControls_In_InputControl
  Initialise : Inport  Port=2
  Bus Selector : BusSelector  OutputSignals=Value,Mode,InitVal,InternalRequest,Inhibit
  LIMPHomePB-Toggle : IOStateMachinesLib/Toggle  InitSource=internal  InitState=InitState  OffStateValue=OffStateValue  OnStateValue=OnStateValue
      settings: SourceProductName=IO State Machines
  InputState : Outport  VectorParamsAs1DForOutWhenUnconnected=off
  wires:
  Initialise/1 -> LIMPHomePB-Toggle/4
  LIMPHomePB-Toggle/1 -> InputState/1
  Bus Selector/5 -> LIMPHomePB-Toggle/6  "<Inhibit>"
  Bus Selector/4 -> LIMPHomePB-Toggle/5  "<InternalRequest>"
  Bus Selector/3 -> LIMPHomePB-Toggle/3  "<InitVal>"
  Bus Selector/2 -> LIMPHomePB-Toggle/2  "<Mode>"
  Bus Selector/1 -> LIMPHomePB-Toggle/1  "<Value>"
  InputControl/1 -> Bus Selector/1

== system IOControls/ForEachVehicle/IOControls/CabControl/DriverDeskLeft/OperatingPanel2/LeftDoorClosePBOperatingPanel2 ==
  note: States:
      | Off
      | On
  InputControl : Inport  OutDataTypeStr=Bus: BD_IOControls_In_InputControl
  Initialise : Inport  Port=2
  Bus Selector : BusSelector  OutputSignals=Value,Mode,InitVal,InternalRequest,Inhibit
  LeftDoorClosePBOperatingPanel2-Momentary : IOStateMachinesLib/Momentary  InitSource=internal  InitState=InitState
      settings: SourceProductName=IO State Machines
  InputState : Outport  VectorParamsAs1DForOutWhenUnconnected=off
  wires:
  Initialise/1 -> LeftDoorClosePBOperatingPanel2-Momentary/4
  LeftDoorClosePBOperatingPanel2-Momentary/1 -> InputState/1
  Bus Selector/5 -> LeftDoorClosePBOperatingPanel2-Momentary/6  "<Inhibit>"
  Bus Selector/4 -> LeftDoorClosePBOperatingPanel2-Momentary/5  "<InternalRequest>"
  Bus Selector/3 -> LeftDoorClosePBOperatingPanel2-Momentary/3  "<InitVal>"
  Bus Selector/2 -> LeftDoorClosePBOperatingPanel2-Momentary/2  "<Mode>"
  Bus Selector/1 -> LeftDoorClosePBOperatingPanel2-Momentary/1  "<Value>"
  InputControl/1 -> Bus Selector/1

== system IOControls/ForEachVehicle/IOControls/CabControl/DriverDeskLeft/OperatingPanel2/LeftDoorOpenPB1OperatingPanel2 ==
  note: States:
      | Off
      | On
  InputControl : Inport  OutDataTypeStr=Bus: BD_IOControls_In_InputControl
  Initialise : Inport  Port=2
  Bus Selector : BusSelector  OutputSignals=Value,Mode,InitVal,InternalRequest,Inhibit
  LeftDoorOpenPB1OperatingPanel2-Momentary : IOStateMachinesLib/Momentary  InitSource=internal  InitState=InitState
      settings: SourceProductName=IO State Machines
  InputState : Outport  VectorParamsAs1DForOutWhenUnconnected=off
  wires:
  Initialise/1 -> LeftDoorOpenPB1OperatingPanel2-Momentary/4
  LeftDoorOpenPB1OperatingPanel2-Momentary/1 -> InputState/1
  Bus Selector/5 -> LeftDoorOpenPB1OperatingPanel2-Momentary/6  "<Inhibit>"
  Bus Selector/4 -> LeftDoorOpenPB1OperatingPanel2-Momentary/5  "<InternalRequest>"
  Bus Selector/3 -> LeftDoorOpenPB1OperatingPanel2-Momentary/3  "<InitVal>"
  Bus Selector/2 -> LeftDoorOpenPB1OperatingPanel2-Momentary/2  "<Mode>"
  Bus Selector/1 -> LeftDoorOpenPB1OperatingPanel2-Momentary/1  "<Value>"
  InputControl/1 -> Bus Selector/1

== system IOControls/ForEachVehicle/IOControls/CabControl/DriverDeskLeft/OperatingPanel2/LeftDoorOpenPBOperatingPanel2 ==
  note: States:
      | Off
      | On
  InputControl : Inport  OutDataTypeStr=Bus: BD_IOControls_In_InputControl
  Initialise : Inport  Port=2
  Bus Selector : BusSelector  OutputSignals=Value,Mode,InitVal,InternalRequest,Inhibit
  LeftDoorOpenPBOperatingPanel2-Momentary : IOStateMachinesLib/Momentary  InitSource=internal  InitState=InitState
      settings: SourceProductName=IO State Machines
  InputState : Outport  VectorParamsAs1DForOutWhenUnconnected=off
  wires:
  Initialise/1 -> LeftDoorOpenPBOperatingPanel2-Momentary/4
  LeftDoorOpenPBOperatingPanel2-Momentary/1 -> InputState/1
  Bus Selector/5 -> LeftDoorOpenPBOperatingPanel2-Momentary/6  "<Inhibit>"
  Bus Selector/4 -> LeftDoorOpenPBOperatingPanel2-Momentary/5  "<InternalRequest>"
  Bus Selector/3 -> LeftDoorOpenPBOperatingPanel2-Momentary/3  "<InitVal>"
  Bus Selector/2 -> LeftDoorOpenPBOperatingPanel2-Momentary/2  "<Mode>"
  Bus Selector/1 -> LeftDoorOpenPBOperatingPanel2-Momentary/1  "<Value>"
  InputControl/1 -> Bus Selector/1

== system IOControls/ForEachVehicle/IOControls/CabControl/DriverDeskLeft/OperatingPanel2/PantoDownPB ==
  note: States:
      | Off
      | On
  InputControl : Inport  OutDataTypeStr=Bus: BD_IOControls_In_InputControl
  Initialise : Inport  Port=2
  Bus Selector : BusSelector  OutputSignals=Value,Mode,InitVal,InternalRequest,Inhibit
  PantoDownPB-Momentary : IOStateMachinesLib/Momentary  InitSource=internal  InitState=InitState
      settings: SourceProductName=IO State Machines
  InputState : Outport  VectorParamsAs1DForOutWhenUnconnected=off
  wires:
  Initialise/1 -> PantoDownPB-Momentary/4
  PantoDownPB-Momentary/1 -> InputState/1
  Bus Selector/5 -> PantoDownPB-Momentary/6  "<Inhibit>"
  Bus Selector/4 -> PantoDownPB-Momentary/5  "<InternalRequest>"
  Bus Selector/3 -> PantoDownPB-Momentary/3  "<InitVal>"
  Bus Selector/2 -> PantoDownPB-Momentary/2  "<Mode>"
  Bus Selector/1 -> PantoDownPB-Momentary/1  "<Value>"
  InputControl/1 -> Bus Selector/1

== system IOControls/ForEachVehicle/IOControls/CabControl/DriverDeskLeft/OperatingPanel2/PantoSelector ==
  note: States:
      | Unit All
      | Unit 3
      | Unit 2
      | Unit 1
  InputControl : Inport  OutDataTypeStr=Bus: BD_IOControls_In_InputControl
  Initialise : Inport  Port=2
  Bus Selector : BusSelector  OutputSignals=Value,Mode,InitVal,InternalRequest,Inhibit
  PantoSelector-Increment : IOStateMachinesLib/Increment  InitSource=internal  InitState=InitState  ControlStates=ControlStates
      settings: SourceProductName=IO State Machines
  InputState : Outport  VectorParamsAs1DForOutWhenUnconnected=off
  wires:
  Initialise/1 -> PantoSelector-Increment/4
  PantoSelector-Increment/1 -> InputState/1
  Bus Selector/5 -> PantoSelector-Increment/6  "<Inhibit>"
  Bus Selector/4 -> PantoSelector-Increment/5  "<InternalRequest>"
  Bus Selector/3 -> PantoSelector-Increment/3  "<InitVal>"
  Bus Selector/2 -> PantoSelector-Increment/2  "<Mode>"
  Bus Selector/1 -> PantoSelector-Increment/1  "<Value>"
  InputControl/1 -> Bus Selector/1

== system IOControls/ForEachVehicle/IOControls/CabControl/DriverDeskLeft/OperatingPanel2/PantoUpPB ==
  note: States:
      | Off
      | On
  InputControl : Inport  OutDataTypeStr=Bus: BD_IOControls_In_InputControl
  Initialise : Inport  Port=2
  Bus Selector : BusSelector  OutputSignals=Value,Mode,InitVal,InternalRequest,Inhibit
  PantoUpPB-Momentary : IOStateMachinesLib/Momentary  InitSource=internal  InitState=InitState
      settings: SourceProductName=IO State Machines
  InputState : Outport  VectorParamsAs1DForOutWhenUnconnected=off
  wires:
  Initialise/1 -> PantoUpPB-Momentary/4
  PantoUpPB-Momentary/1 -> InputState/1
  Bus Selector/5 -> PantoUpPB-Momentary/6  "<Inhibit>"
  Bus Selector/4 -> PantoUpPB-Momentary/5  "<InternalRequest>"
  Bus Selector/3 -> PantoUpPB-Momentary/3  "<InitVal>"
  Bus Selector/2 -> PantoUpPB-Momentary/2  "<Mode>"
  Bus Selector/1 -> PantoUpPB-Momentary/1  "<Value>"
  InputControl/1 -> Bus Selector/1

== system IOControls/ForEachVehicle/IOControls/CabControl/DriverDeskLeft/OperatingPanel2/PowerOffPB ==
  note: States:
      | Off
      | On
  InputControl : Inport  OutDataTypeStr=Bus: BD_IOControls_In_InputControl
  Initialise : Inport  Port=2
  Bus Selector : BusSelector  OutputSignals=Value,Mode,InitVal,InternalRequest,Inhibit
  PowerOffPB-Momentary : IOStateMachinesLib/Momentary  InitSource=internal  InitState=InitState
      settings: SourceProductName=IO State Machines
  InputState : Outport  VectorParamsAs1DForOutWhenUnconnected=off
  wires:
  Initialise/1 -> PowerOffPB-Momentary/4
  PowerOffPB-Momentary/1 -> InputState/1
  Bus Selector/5 -> PowerOffPB-Momentary/6  "<Inhibit>"
  Bus Selector/4 -> PowerOffPB-Momentary/5  "<InternalRequest>"
  Bus Selector/3 -> PowerOffPB-Momentary/3  "<InitVal>"
  Bus Selector/2 -> PowerOffPB-Momentary/2  "<Mode>"
  Bus Selector/1 -> PowerOffPB-Momentary/1  "<Value>"
  InputControl/1 -> Bus Selector/1

== system IOControls/ForEachVehicle/IOControls/CabControl/DriverDeskLeft/OperatingPanel2/SafetyCutoutSS ==
  note: States:
      | Normal
      | Cutout
  InputControl : Inport  OutDataTypeStr=Bus: BD_IOControls_In_InputControl
  Initialise : Inport  Port=2
  Bus Selector : BusSelector  OutputSignals=Value,Mode,InitVal,InternalRequest,Inhibit
  SafetyCutoutSS-Toggle : IOStateMachinesLib/Toggle  InitSource=internal  InitState=InitState  OffStateValue=OffStateValue  OnStateValue=OnStateValue
      settings: SourceProductName=IO State Machines
  InputState : Outport  VectorParamsAs1DForOutWhenUnconnected=off
  wires:
  Initialise/1 -> SafetyCutoutSS-Toggle/4
  SafetyCutoutSS-Toggle/1 -> InputState/1
  Bus Selector/5 -> SafetyCutoutSS-Toggle/6  "<Inhibit>"
  Bus Selector/4 -> SafetyCutoutSS-Toggle/5  "<InternalRequest>"
  Bus Selector/3 -> SafetyCutoutSS-Toggle/3  "<InitVal>"
  Bus Selector/2 -> SafetyCutoutSS-Toggle/2  "<Mode>"
  Bus Selector/1 -> SafetyCutoutSS-Toggle/1  "<Value>"
  InputControl/1 -> Bus Selector/1
